simulink model "simulink_daq_module_win"  (Simulink 7.4)
settings: Solver=FixedStepDiscrete  StartTime=0.0  StopTime=inf  FixedStep=1/2400  RelTol=1e-3
libraries: dspsigops x3, dspbuff3 x3
settings Model: Creator=breidi  LastModifiedBy=breidi
settings SolverCC: InsertRTBMode=Never (minimum delay)
settings OptimizationCC: InlineParams=on  InlineInvariantSignals=on  EnhancedBackFolding=on  EfficientFloat2IntCast=on  SimCompilerOptimization=On
settings HardwareCC: ProdIntDivRoundTo=Zero  ProdEndianess=LittleEndian  ProdHWDeviceType=Generic->32-bit x86 compatible
settings RTWCC: ProcessScript=grt_make_rtw_hook  TargetLang=C++  RTWCompilerOptimization=On
settings CodeAppCC: MaxIdLength=95

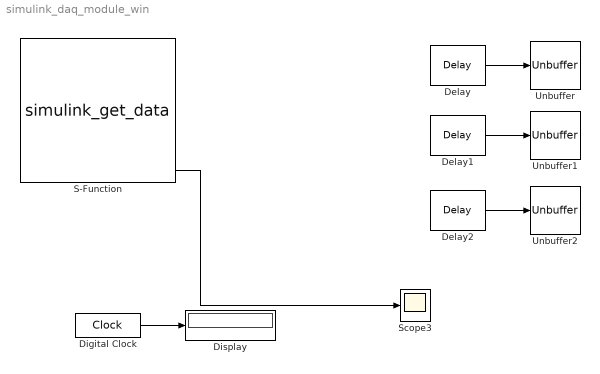
== system simulink_daq_module_win ==
  Delay : dspsigops/Delay  dly_unit=Samples  delay=0  ic_detail=off  dif_ic_for_ch=off  dif_ic_for_dly=off  ic=0  reset_popup=None
  Delay1 : dspsigops/Delay  dly_unit=Samples  delay=0  ic_detail=off  dif_ic_for_ch=off  dif_ic_for_dly=off  ic=0  reset_popup=None
  Delay2 : dspsigops/Delay  dly_unit=Samples  delay=0  ic_detail=off  dif_ic_for_ch=off  dif_ic_for_dly=off  ic=0  reset_popup=None
  Digital Clock : DigitalClock
  Display : Display
  S-Function : S-Function  Priority=1  FunctionName=simulink_get_data  Parameters=master_info, sig_info, ch_info, server_info  EnableBusSupport=off  mask{ip='127.0.0.1', port=9000, proto='tcp'}
      mask prompts: ip "Server IP"; proto "Protocol"
      mask init:
      | global master_info;
      | global sig_info;
      | global ch_info;
      | global fs;
      | 
      | fs = 0;
      | bs = 0;
      | 
      | [master_info sig_info ch_info server_info_tmp] = mex_get_config(ip, port, proto);
      | server_info{1} = proto;
      | server_info{2} = ip;
      | server_info{3} = server_info_tmp;
      | 
      | disp(' ');
      | disp(' ----------------------------------------------------------------------------------------------------- ');
      | disp(' ');
      | disp(' ***** NOTICE: Initialization done in "Net Signal Client" -> Edit Mask -> Initialization! ***** ');
      | 
      | disp(' ');
      | disp('SignalServer Information (protocol, server-IP, server-port):');
      | disp(server_info);
      | 
      | disp(' ');
      | disp('Master Sampling Rate and Blocksize:');
      | disp(master_info);
      | disp('Signal Types Info:  (Flag, Type, BS, NrCh, Fs)');
      | disp(sig_info);
      | disp('Channel Info:  (Name, Type)');
      | disp(ch_info);
      | disp(' ');
      | 
      | fs = master_info(1);
      | bs = master_info(2);
      | 
      | % for n = 1:size(sig_info,1)
      | % %   port_label('output', 1, num2str(cell2mat(sig_info(n,2))) );
      | % end
      | % port_label('input', 1, 'a');
      | % num2str(cell2mat(sig_info(n,2)))
      | 
      | set_param(gcs, 'SolverName', 'FixedStepDiscrete');
      | set_param(gcs, 'FixedStep', [ num2str(1) '/' num2str(fs)])
      | 
      | % set_param(gcs, 'SolverMode', 'Auto');
      | % set_param(gcs, 'FixedStep', '1');
      mask Display:
      | disp('TOBI Signal\nClient')
      | port_label('output', 1, num2str(cell2mat(sig_info(1,2))) );
      | port_label('output', size(sig_info,1)+1, 'events' );
      | port_label('output', size(sig_info,1)+2, 'sample nr' );
      | port_label('output', size(sig_info,1)+3, 'timestamp' );
      | port_label('output', size(sig_info,1)+4, 'sys/sim time' );
  Scope3 : Scope
      settings: YMin=-0.025  YMax=0.175  SaveName=ScopeData3
  Unbuffer : dspbuff3/Unbuffer  ic=0
  Unbuffer1 : dspbuff3/Unbuffer  ic=0
  Unbuffer2 : dspbuff3/Unbuffer  ic=0
  wires:
  Digital Clock/1 -> Display/1
  Delay/1 -> Unbuffer/1
  Delay1/1 -> Unbuffer1/1
  Delay2/1 -> Unbuffer2/1
  S-Function/5 -> Scope3/1
